simulink model "vhull"  (Simulink 7.5)
settings: Solver=ode45  StartTime=0.0  StopTime=10.0  RelTol=1e-3
values from neighbouring files (symbols this model uses):
  a1 = 5    [valuables.m]
  a2 = 2*a1    (= 10)    [valuables.m]
  b = 3.7/2    (= 1.85)    [valuables.m]
settings Model: Creator=ex08148  LastModifiedBy=ex08148

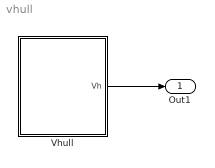
== system vhull ==
  Vhull : Subsystem
  Out1 : Outport  OutDataType=sfix(16)  OutScaling=2^0
  wires:
  Vhull/1(Vh) -> Out1/1

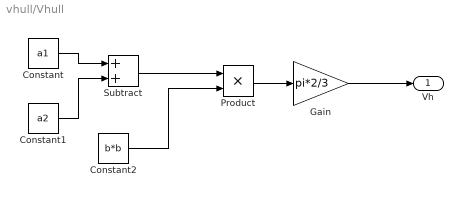
== system vhull/Vhull ==
  Constant : Constant  Value=a1  OutDataType=sfix(16)  OutScaling=2^0
  Constant1 : Constant  Value=a2  OutDataType=sfix(16)  OutScaling=2^0
  Constant2 : Constant  Value=b*b  OutDataType=sfix(16)  OutScaling=2^0
  Gain : Gain  Gain=pi*2/3  ParameterDataType=sfix(16)  ParameterScaling=2^0  OutDataType=sfix(16)  OutScaling=2^0
  Product : Product  OutDataType=sfix(16)  OutScaling=2^0  RndMeth=Zero
  Subtract : Sum  OutDataType=sfix(16)  OutScaling=2^-10
  Vh : Outport  OutDataType=sfix(16)  OutScaling=2^0
  wires:
  Constant/1 -> Subtract/1
  Constant1/1 -> Subtract/2
  Subtract/1 -> Product/1
  Constant2/1 -> Product/2
  Product/1 -> Gain/1
  Gain/1 -> Vh/1
